simulink library "Battery7"  (R2024b)
settings: Solver=VariableStepAuto  StartTime=0.0  StopTime=10.0  RelTol=1e-3
undefined symbols (not defined in the file or in its folder): battery_builder_rtmsupport, gcbh
libraries: nesl_utility x2, Battery7_lib x2
settings Model: Creator=yeswa  LastModifiedBy=yeswa

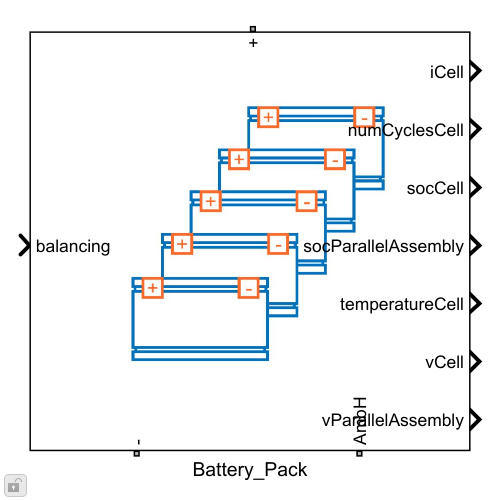
[thumbnail: Simulink's stored preview of the top-level diagram]
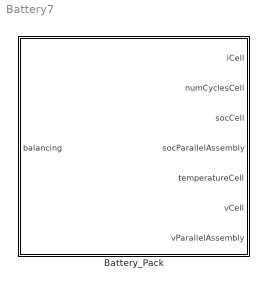
== system Battery7 ==
  Battery_Pack : Subsystem  LoadFcn=battery_builder_rtmsupport('loadfcn',gcbh);
      settings: CopyFcn=battery_builder_rtmsupport('copyfcn',gcbh);  PreCopyFcn=battery_builder_rtmsupport('precopyfcn',gcbh);  PreDeleteFcn=battery_builder_rtmsupport('predeletefcn',gcbh);  PortSchema="{\"entries\":[{\"content\":{\"sides\":[{\"content\":{\"connectorIds\":[\"LConn1\"]},\"type\":\"ConnectorPlacement.EquallySpacedRectSide\",\"uuid\":\"4692a778-4fa6-4ab6-bac3-76305c043af6\"},{\"content\":{\"connectorIds\":[\"RConn1\",\"RConn2\"],\"side\":\"RIGHT\"},\"type\":\"ConnectorPlacement.EquallySpacedRectSide\",\"uuid\":\"f98963b2-f24c-4446-9753-78469fdf523d\"},{\"content\":{\"connectorIds\":[\"In1\"],\"side\":\"TOP\"},\"type\":\"ConnectorPlacement.EquallySpacedRectSide\",\"uuid\":\"d3c31044-be3d-42c0-914f-e8152f50e02f\"},{\"content\":{\"connectorIds\":[\"Out1\",\"Out2\",\"Out3\",\"Out4\",\"Out5\",\"Out6\",\"Out7\"],\"side\":\"BOTTOM\"},\"type\":\"ConnectorPlacement.EquallySpacedRectSide\",\"uuid\":\"97db5bca-7031-400f-85b4-629ab66f98c2\"}]},\"type\":\"ConnectorPlacement.EquallySpacedConnector\",\"uuid\":\"5f8ad85d-1982-46fd-b866-406ee9ad9b25\"}],\"packageUris\":[\"http://schema.mathworks.com/mf0/Connector/R2020b\"],\"version\":\"1.0\"}"
      mask Display: image('$imagefile')

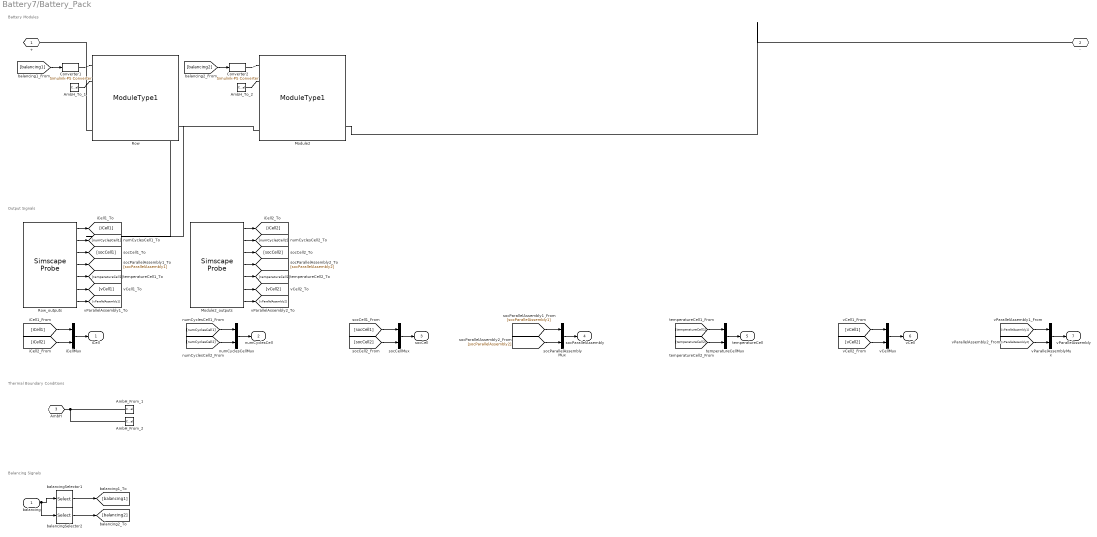
== system Battery7/Battery_Pack ==
  note: Battery Modules
  note: Output Signals
  note: Thermal Boundary Conditions
  note: Balancing Signals
  balancing : Inport  PortDimensions=16
  AmbH_From_1 : ConnectionLabel  Label=ambH_1
  AmbH_From_2 : ConnectionLabel  Label=ambH_2
  AmbH_To_1 : ConnectionLabel  Label=ambH_1
  AmbH_To_2 : ConnectionLabel  Label=ambH_2
  Converter1 : nesl_utility/Simulink-PS Converter  PhysicalDomain=network_engine_domain  SubClassName=ps_input  LeftPortType=input  RightPortType=output  PseudoPeriodic=off  Frequencies=[]  NoiseDistribution=none  NoiseParameters=[]  Unit=1  AffineConversion=off  FilteringAndDerivatives=provide  SimscapeFilterOrder=1  InputFilterTimeConstant=0.001  UdotUserProvided=0
  Converter2 : nesl_utility/Simulink-PS Converter  PhysicalDomain=network_engine_domain  SubClassName=ps_input  LeftPortType=input  RightPortType=output  PseudoPeriodic=off  Frequencies=[]  NoiseDistribution=none  NoiseParameters=[]  Unit=1  AffineConversion=off  FilteringAndDerivatives=provide  SimscapeFilterOrder=1  InputFilterTimeConstant=0.001  UdotUserProvided=0
  Module2 : Battery7_lib/Modules/ModuleType1  SOC_vecCell=ModuleType1.SOC_vecCell  T_vecCell=ModuleType1.T_vecCell K  V0_matCell=ModuleType1.V0_matCell V  V_rangeCell=ModuleType1.V_rangeCell V  R0_matCell=ModuleType1.R0_matCell Ohm  AHCell=ModuleType1.AHCell A*hr  extrapolation_optionCell=simscape.enum.extrapolation.nearest  R1_matCell=ModuleType1.R1_matCell Ohm  tau1_matCell=ModuleType1.tau1_matCell s  R2_matCell=ModuleType1.R2_matCell Ohm  tau2_matCell=ModuleType1.tau2_matCell s  R3_matCell=ModuleType1.R3_matCell Ohm  tau3_matCell=ModuleType1.tau3_matCell s  thermal_massCell=ModuleType1.thermal_massCell J/K  AmbientResistance=ModuleType1.AmbientResistance K/W  XminThermalResistance=ModuleType1.XminThermalResistance K/W  XmaxThermalResistance=ModuleType1.XmaxThermalResistance K/W  YminThermalResistance=ModuleType1.YminThermalResistance K/W  YmaxThermalResistance=ModuleType1.YmaxThermalResistance K/W  CellBalancingClosedResistance=ModuleType1.CellBalancingClosedResistance Ohm  CellBalancingOpenConductance=ModuleType1.CellBalancingOpenConductance 1/Ohm  CellBalancingThreshold=ModuleType1.CellBalancingThreshold  CellBalancingResistance=ModuleType1.CellBalancingResistance Ohm  P=1  S=8  NumXminConnections=8  XminConnectionsMapping=[1, 2, 3, 4, 5, 6, 7, 8]  NumCellsAtXminBoundary=8  CellsInModelAtXminBoundary=[1, 1, 1, 1, 1, 1, 1, 1]  NumXmaxConnections=8  XmaxConnectionsMapping=[1, 2, 3, 4, 5, 6, 7, 8]  NumCellsAtXmaxBoundary=8  CellsInModelAtXmaxBoundary=[1, 1, 1, 1, 1, 1, 1, 1]  NumYminConnections=1  YminConnectionsMapping=1  NumCellsAtYminBoundary=1  CellsInModelAtYminBoundary=1  NumYmaxConnections=1  YmaxConnectionsMapping=8  NumCellsAtYmaxBoundary=1  CellsInModelAtYmaxBoundary=1  SeriesGrouping=[1, 1, 1, 1, 1, 1, 1, 1]  ParallelGrouping=[1, 1, 1, 1, 1, 1, 1, 1]  iCell_specify=on  iCell_priority=None  iCell=Module2.iCell A  iCell_nominal_specify=off  iCell_nominal_value=1  iCell_nominal_unit=A  vCell_specify=on  vCell_priority=None  vCell=Module2.vCell V  vCell_nominal_specify=off  vCell_nominal_value=1  vCell_nominal_unit=V  socCell_specify=on  socCell_priority=High  socCell=Module2.socCell  socCell_nominal_specify=off  socCell_nominal_value=1  socCell_nominal_unit=1  numCyclesCell_specify=on  numCyclesCell_priority=High  numCyclesCell=Module2.numCyclesCell  numCyclesCell_nominal_specify=off  numCyclesCell_nominal_value=1  numCyclesCell_nominal_unit=1  temperatureCell_specify=on  temperatureCell_priority=High  temperatureCell=Module2.temperatureCell K  temperatureCell_nominal_specify=off  temperatureCell_nominal_value=1  temperatureCell_nominal_unit=K  vParallelAssembly_specify=on  vParallelAssembly_priority=None  vParallelAssembly=Module2.vParallelAssembly V  vParallelAssembly_nominal_specify=off  vParallelAssembly_nominal_value=1  vParallelAssembly_nominal_unit=V  socParallelAssembly_specify=on  socParallelAssembly_priority=None  socParallelAssembly=Module2.socParallelAssembly  socParallelAssembly_nominal_specify=off  socParallelAssembly_nominal_value=1  socParallelAssembly_nominal_unit=1
      settings: InternalSimscapePortConfiguration="{\"Bottom\":[{\"id\":\"n\",\"label\":\"-\",\"type\":\"foundation.electrical.electrical\"}],\"Left\":[{\"id\":\"enableCellBalancing\",\"label\":\"CB\",\"type\":\"input\"},{\"id\":\"AmbH\",\"label\":\"AmbH\",\"type\":\"foundation.thermal.thermal\"},{\"id\":\"XminH\",\"label\":\"XminH\",\"type\":\"foundation.thermal.thermal\"},{\"id\":\"YminH\",\"label\":\"YminH\",\"type\":\"foundation.thermal.thermal\"}],\"Right\":[{\"id\":\"XmaxH\",\"label\":\"XmaxH\",\"type\":\"foundation.thermal.thermal\"},{\"id\":\"YmaxH\",\"label\":\"YmaxH\",\"type\":\"foundation.thermal.thermal\"}],\"Top\":[{\"id\":\"p\",\"label\":\"+\",\"type\":\"foundation.electrical.electrical\"}]}"
  Module2_outputs : SimscapeProbe  BoundBlock=3  Variables="{\"iCell\":{\"Unit\":\"A\",\"PortLabel\":\"iCell\",\"Probing\":\"ON\"},\"numCyclesCell\":{\"Unit\":\"1\",\"PortLabel\":\"numCyclesCell\",\"Probing\":\"ON\"},\"socCell\":{\"Unit\":\"1\",\"PortLabel\":\"socCell\",\"Probing\":\"ON\"},\"socParallelAssembly\":{\"Unit\":\"1\",\"PortLabel\":\"socParallelAssembly\",\"Probing\":\"ON\"},\"temperatureCell\":{\"Unit\":\"K\",\"PortLabel\":\"temperatureCell\",\"Probing\":\"ON\"},\"vCell\":{\"Unit\":\"V\",\"PortLabel\":\"vCell\",\"Probing\":\"ON\"},\"vParallelAssembly\":{\"Unit\":\"V\",\"PortLabel\":\"vParallelAssembly\",\"Probing\":\"ON\"}}"
  Row : Battery7_lib/Modules/ModuleType1  SOC_vecCell=ModuleType1.SOC_vecCell  T_vecCell=ModuleType1.T_vecCell K  V0_matCell=ModuleType1.V0_matCell V  V_rangeCell=ModuleType1.V_rangeCell V  R0_matCell=ModuleType1.R0_matCell Ohm  AHCell=ModuleType1.AHCell A*hr  extrapolation_optionCell=simscape.enum.extrapolation.nearest  R1_matCell=ModuleType1.R1_matCell Ohm  tau1_matCell=ModuleType1.tau1_matCell s  R2_matCell=ModuleType1.R2_matCell Ohm  tau2_matCell=ModuleType1.tau2_matCell s  R3_matCell=ModuleType1.R3_matCell Ohm  tau3_matCell=ModuleType1.tau3_matCell s  thermal_massCell=ModuleType1.thermal_massCell J/K  AmbientResistance=ModuleType1.AmbientResistance K/W  XminThermalResistance=ModuleType1.XminThermalResistance K/W  XmaxThermalResistance=ModuleType1.XmaxThermalResistance K/W  YminThermalResistance=ModuleType1.YminThermalResistance K/W  YmaxThermalResistance=ModuleType1.YmaxThermalResistance K/W  CellBalancingClosedResistance=ModuleType1.CellBalancingClosedResistance Ohm  CellBalancingOpenConductance=ModuleType1.CellBalancingOpenConductance 1/Ohm  CellBalancingThreshold=ModuleType1.CellBalancingThreshold  CellBalancingResistance=ModuleType1.CellBalancingResistance Ohm  P=1  S=8  NumXminConnections=8  XminConnectionsMapping=[1, 2, 3, 4, 5, 6, 7, 8]  NumCellsAtXminBoundary=8  CellsInModelAtXminBoundary=[1, 1, 1, 1, 1, 1, 1, 1]  NumXmaxConnections=8  XmaxConnectionsMapping=[1, 2, 3, 4, 5, 6, 7, 8]  NumCellsAtXmaxBoundary=8  CellsInModelAtXmaxBoundary=[1, 1, 1, 1, 1, 1, 1, 1]  NumYminConnections=1  YminConnectionsMapping=1  NumCellsAtYminBoundary=1  CellsInModelAtYminBoundary=1  NumYmaxConnections=1  YmaxConnectionsMapping=8  NumCellsAtYmaxBoundary=1  CellsInModelAtYmaxBoundary=1  SeriesGrouping=[1, 1, 1, 1, 1, 1, 1, 1]  ParallelGrouping=[1, 1, 1, 1, 1, 1, 1, 1]  iCell_specify=on  iCell_priority=None  iCell=Row.iCell A  iCell_nominal_specify=off  iCell_nominal_value=1  iCell_nominal_unit=A  vCell_specify=on  vCell_priority=None  vCell=Row.vCell V  vCell_nominal_specify=off  vCell_nominal_value=1  vCell_nominal_unit=V  socCell_specify=on  socCell_priority=High  socCell=Row.socCell  socCell_nominal_specify=off  socCell_nominal_value=1  socCell_nominal_unit=1  numCyclesCell_specify=on  numCyclesCell_priority=High  numCyclesCell=Row.numCyclesCell  numCyclesCell_nominal_specify=off  numCyclesCell_nominal_value=1  numCyclesCell_nominal_unit=1  temperatureCell_specify=on  temperatureCell_priority=High  temperatureCell=Row.temperatureCell K  temperatureCell_nominal_specify=off  temperatureCell_nominal_value=1  temperatureCell_nominal_unit=K  vParallelAssembly_specify=on  vParallelAssembly_priority=None  vParallelAssembly=Row.vParallelAssembly V  vParallelAssembly_nominal_specify=off  vParallelAssembly_nominal_value=1  vParallelAssembly_nominal_unit=V  socParallelAssembly_specify=on  socParallelAssembly_priority=None  socParallelAssembly=Row.socParallelAssembly  socParallelAssembly_nominal_specify=off  socParallelAssembly_nominal_value=1  socParallelAssembly_nominal_unit=1
      settings: InternalSimscapePortConfiguration="{\"Bottom\":[{\"id\":\"n\",\"label\":\"-\",\"type\":\"foundation.electrical.electrical\"}],\"Left\":[{\"id\":\"enableCellBalancing\",\"label\":\"CB\",\"type\":\"input\"},{\"id\":\"AmbH\",\"label\":\"AmbH\",\"type\":\"foundation.thermal.thermal\"},{\"id\":\"XminH\",\"label\":\"XminH\",\"type\":\"foundation.thermal.thermal\"},{\"id\":\"YminH\",\"label\":\"YminH\",\"type\":\"foundation.thermal.thermal\"}],\"Right\":[{\"id\":\"XmaxH\",\"label\":\"XmaxH\",\"type\":\"foundation.thermal.thermal\"},{\"id\":\"YmaxH\",\"label\":\"YmaxH\",\"type\":\"foundation.thermal.thermal\"}],\"Top\":[{\"id\":\"p\",\"label\":\"+\",\"type\":\"foundation.electrical.electrical\"}]}"
  Row_outputs : SimscapeProbe  BoundBlock=2  Variables="{\"iCell\":{\"Unit\":\"A\",\"PortLabel\":\"iCell\",\"Probing\":\"ON\"},\"numCyclesCell\":{\"Unit\":\"1\",\"PortLabel\":\"numCyclesCell\",\"Probing\":\"ON\"},\"socCell\":{\"Unit\":\"1\",\"PortLabel\":\"socCell\",\"Probing\":\"ON\"},\"socParallelAssembly\":{\"Unit\":\"1\",\"PortLabel\":\"socParallelAssembly\",\"Probing\":\"ON\"},\"temperatureCell\":{\"Unit\":\"K\",\"PortLabel\":\"temperatureCell\",\"Probing\":\"ON\"},\"vCell\":{\"Unit\":\"V\",\"PortLabel\":\"vCell\",\"Probing\":\"ON\"},\"vParallelAssembly\":{\"Unit\":\"V\",\"PortLabel\":\"vParallelAssembly\",\"Probing\":\"ON\"}}"
  balancingSelector1 : Selector  InputPortWidth=16  IndexOptions=Index vector (dialog)  Indices="[1  2  3  4  5  6  7  8]"  OutputSizes=1
  balancingSelector2 : Selector  InputPortWidth=16  IndexOptions=Index vector (dialog)  Indices="[9  10  11  12  13  14  15  16]"  OutputSizes=1
  iCellMux : Mux  Inputs=2
  numCyclesCellMux : Mux  Inputs=2
  socCellMux : Mux  Inputs=2
  socParallelAssemblyMux : Mux  Inputs=2
  temperatureCellMux : Mux  Inputs=2
  vCellMux : Mux  Inputs=2
  vParallelAssemblyMux : Mux  Inputs=2
  + : PMIOPort  Side=Left
  - : PMIOPort  Port=2  Side=Right
  AmbH : PMIOPort  Port=3  Side=Right  ConnectionType=Connection: foundation.thermal.thermal
  iCell : Outport
  numCyclesCell : Outport  Port=2
  socCell : Outport  Port=3
  socParallelAssembly : Outport  Port=4
  temperatureCell : Outport  Port=5
  vCell : Outport  Port=6
  vParallelAssembly : Outport  Port=7
  wires:
  Row_outputs/1 -> [iCell1]
  iCellMux/1 -> iCell/1
  [iCell1] -> iCellMux/1
  Row_outputs/2 -> [numCyclesCell1]
  numCyclesCellMux/1 -> numCyclesCell/1
  [numCyclesCell1] -> numCyclesCellMux/1
  Row_outputs/3 -> [socCell1]
  socCellMux/1 -> socCell/1
  [socCell1] -> socCellMux/1
  Row_outputs/4 -> [socParallelAssembly1]
  socParallelAssemblyMux/1 -> socParallelAssembly/1
  [socParallelAssembly1] -> socParallelAssemblyMux/1
  Row_outputs/5 -> [temperatureCell1]
  temperatureCellMux/1 -> temperatureCell/1
  [temperatureCell1] -> temperatureCellMux/1
  Row_outputs/6 -> [vCell1]
  vCellMux/1 -> vCell/1
  [vCell1] -> vCellMux/1
  Row_outputs/7 -> [vParallelAssembly1]
  vParallelAssemblyMux/1 -> vParallelAssembly/1
  [vParallelAssembly1] -> vParallelAssemblyMux/1
  Module2_outputs/1 -> [iCell2]
  [iCell2] -> iCellMux/2
  Module2_outputs/2 -> [numCyclesCell2]
  [numCyclesCell2] -> numCyclesCellMux/2
  Module2_outputs/3 -> [socCell2]
  [socCell2] -> socCellMux/2
  Module2_outputs/4 -> [socParallelAssembly2]
  [socParallelAssembly2] -> socParallelAssemblyMux/2
  Module2_outputs/5 -> [temperatureCell2]
  [temperatureCell2] -> temperatureCellMux/2
  Module2_outputs/6 -> [vCell2]
  [vCell2] -> vCellMux/2
  Module2_outputs/7 -> [vParallelAssembly2]
  [vParallelAssembly2] -> vParallelAssemblyMux/2
  [balancing1] -> Converter1/1
  balancing/1 -> balancingSelector1/1, balancingSelector2/1
  balancingSelector1/1 -> [balancing1]
  [balancing2] -> Converter2/1
  balancingSelector2/1 -> [balancing2]
  connections:
  Module2/LConn5 -- Row/RConn3
  Row/LConn5 -- +/RConn1
  Module2/RConn3 -- -/RConn1
  Converter1/RConn1 -- Row/LConn1
  Converter2/RConn1 -- Module2/LConn1
  AmbH_To_1/LConn1 -- Row/LConn2
  AmbH/RConn1 -- AmbH_From_1/LConn1 -- AmbH_From_2/LConn1
  AmbH_To_2/LConn1 -- Module2/LConn2
